simulink model "nonliear_EHA"  (R2023a)
settings: Solver=VariableStepAuto  StartTime=0.0  StopTime=15  RelTol=1e-3
undefined symbols (not defined in the file): Ap, Ba, Bcs, Be, Jcs, Kf, Ki, Kl, Kp, Kv, Lm, Td, Tn, Tv, Vo, Wd1, Wff, Wn, Wv
libraries: simulink x2
settings Model: LastModifiedBy=asans

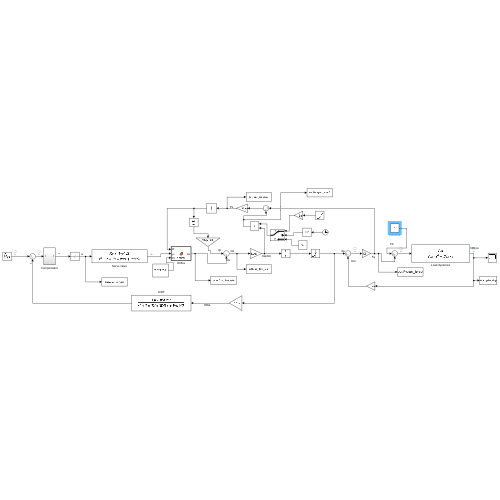
[thumbnail: Simulink's stored preview of the top-level diagram]
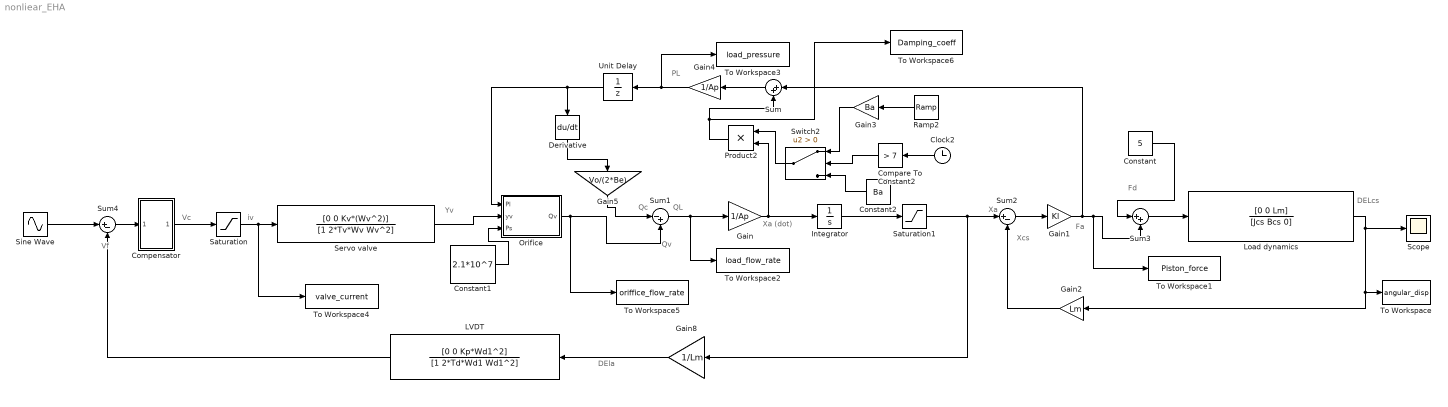
== system nonliear_EHA ==
  note: DEla
  note: DELcs
  note: Fd
  note: Fa
  note: Xcs
  note: Xa
  note: PL
  note: Xa (dot)
  note: QL
  note: Qc
  note: Qv
  note: Yv
  note: iv
  note: Vc
  note: Vf
  Clock2 : Clock
  Compare To Constant2 : simulink/Logic and Bit Operations/Compare To Constant  relop=>  const=7  OutDataTypeStr=boolean
  Compensator : Subsystem
  Constant : Constant  Value=5
  Constant1 : Constant  Value=2.1*10^7
  Constant2 : Constant  Value=Ba
  Derivative : Derivative
  Gain : Gain  Gain=1/Ap
  Gain1 : Gain  Gain=Kl
  Gain2 : Gain  Gain=Lm
  Gain3 : Gain  Gain=Ba
  Gain4 : Gain  Gain=1/Ap
  Gain5 : Gain  Gain=Vo/(2*Be)
  Gain8 : Gain  Gain=1/Lm
  Integrator : Integrator
  LVDT : TransferFcn  Numerator=[0 0 Kp*Wd1^2]  Denominator=[1 2*Td*Wd1 Wd1^2]
  Load dynamics : TransferFcn  Numerator=[0 0 Lm]  Denominator=[Jcs Bcs 0]
  Orifice : MATLAB Function  TreatAsAtomicUnit=on
  Product2 : Product
  Ramp2 : simulink/Sources/Ramp  slope=-1.5  start=0  InitialOutput=0
  Saturation : Saturate
  Saturation1 : Saturate
  Scope : Scope
  Servo valve : TransferFcn  Numerator=[0 0 Kv*(Wv^2)]  Denominator=[1 2*Tv*Wv Wv^2]
  Sine Wave : Sin  Amplitude=9  SampleTime=0
  Sum : Sum  Inputs=|++
  Sum1 : Sum  Inputs=|-+
  Sum2 : Sum  Inputs=|+-
  Sum3 : Sum  Inputs=|++
  Sum4 : Sum  Inputs=|+-
  Switch2 : Switch  Criteria=u2 > Threshold  SaturateOnIntegerOverflow=off  InputSameDT=off
  To Workspace : ToWorkspace  VariableName=angular_disp  SaveFormat=Timeseries  SampleTime=-1
  To Workspace1 : ToWorkspace  VariableName=Piston_force  SaveFormat=Timeseries  SampleTime=-1
  To Workspace2 : ToWorkspace  VariableName=load_flow_rate  SaveFormat=Timeseries  SampleTime=-1
  To Workspace3 : ToWorkspace  VariableName=load_pressure  SaveFormat=Timeseries  SampleTime=-1
  To Workspace4 : ToWorkspace  VariableName=valve_current  SaveFormat=Timeseries  SampleTime=-1
  To Workspace5 : ToWorkspace  VariableName=oriffice_flow_rate  SaveFormat=Timeseries  SampleTime=-1
  To Workspace6 : ToWorkspace  VariableName=Damping_coeff  SaveFormat=Timeseries  SampleTime=-1
  Unit Delay : UnitDelay  SampleTime=-1  HasFrameUpgradeWarning=on
  wires:
  Sum4/1 -> Compensator/1(In1)
  Compensator/1(Out1) -> Saturation/1
  Saturation/1 -> To Workspace4/1, Servo valve/1
  Servo valve/1 -> Orifice/2(yv)
  Orifice/1(Qv) -> To Workspace5/1, Sum1/2
  Integrator/1 -> Saturation1/1
  Saturation1/1 -> Gain8/1, Sum2/1
  Sum2/1 -> Gain1/1
  Sum3/1 -> Load dynamics/1
  Load dynamics/1 -> Gain2/1, To Workspace/1, Scope/1
  Gain2/1 -> Sum2/2
  Sum/1 -> Gain4/1
  Gain8/1 -> LVDT/1
  LVDT/1 -> Sum4/2
  Derivative/1 -> Gain5/1
  Gain5/1 -> Sum1/1
  Constant1/1 -> Orifice/3(Ps)
  Constant/1 -> Sum3/1
  Sum1/1 -> To Workspace2/1, Gain/1
  Gain1/1 -> Sum/1, To Workspace1/1, Sum3/2
  Gain4/1 -> To Workspace3/1, Unit Delay/1
  Unit Delay/1 -> Orifice/1(Pl), Derivative/1
  Sine Wave/1 -> Sum4/1
  Gain/1 -> Integrator/1, Product2/2
  Switch2/1 -> Product2/1
  Clock2/1 -> Compare To Constant2/1
  Ramp2/1 -> Gain3/1
  Gain3/1 -> Switch2/1
  Compare To Constant2/1 -> Switch2/2
  Constant2/1 -> Switch2/3
  Product2/1 -> Sum/2, To Workspace6/1

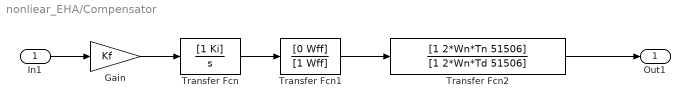
== system nonliear_EHA/Compensator ==
  In1 : Inport
  Gain : Gain  Gain=Kf
  Transfer Fcn : TransferFcn  Numerator=[1 Ki]  Denominator=[1 0]
  Transfer Fcn1 : TransferFcn  Numerator=[0 Wff]  Denominator=[1 Wff]
  Transfer Fcn2 : TransferFcn  Numerator=[1 2*Wn*Tn 51506]  Denominator=[1 2*Wn*Td 51506]
  Out1 : Outport
  wires:
  In1/1 -> Gain/1
  Transfer Fcn2/1 -> Out1/1
  Transfer Fcn1/1 -> Transfer Fcn2/1
  Transfer Fcn/1 -> Transfer Fcn1/1
  Gain/1 -> Transfer Fcn/1

== matlab function nonliear_EHA/Orifice ==
  data: Pl input; Qv output; yv input; Ps input
function Qv = orifice(Pl, yv, Ps)
gm =sign(yv);sig=0.5e-6;del=0.5e-6;Kfn=2.386e-4;Cr=0.5e-6;
xv=yv-del*(1-exp(-sig*abs(yv)/Cr/del))*gm;
Qv=Kfn*xv*sqrt(abs(Ps-gm*Pl))*sign(Ps-gm*Pl);
